simulink model "robosimulador"  (R2021b)
settings: Solver=VariableStepAuto  StartTime=0.0  StopTime=Time(length(Time))  MaxStep=1e-3  RelTol=1e-3
model workspace: external: MATLAB File /home/fabio/Desktop/Larc 2021/robosimulador_DataFile.m (data not in the file)
values from neighbouring files (symbols this model uses):
  j = length(Q)    [Cinematica_Comb.m]    (also in Cinematica_Heli_Coronal.m; Cinematica_Heli_Direta_Coronal.m; Cinematica_Heli_Sagital.m)
  Q = Qr    [Cinematica_Comb.m]
  X = zeros(1,14)    [Cinematica_Comb.m]    (also in Cinematica_Heli_Coronal.m = zeros(1,6); Cinematica_Heli_Direta_Coronal.m = zeros(1,6); Cinematica_Heli_Sagital.m = zeros(1,8))
  Y = zeros(1,14)    [Cinematica_Comb.m]    (also in Cinematica_Heli_Coronal.m = zeros(1,6); Cinematica_Heli_Direta_Coronal.m = zeros(1,6); Cinematica_Heli_Sagital.m = zeros(1,8))
  Z = zeros(1,14)    [Cinematica_Comb.m]    (also in Cinematica_Heli_Coronal.m = zeros(1,6); Cinematica_Heli_Direta_Coronal.m = zeros(1,6); Cinematica_Heli_Sagital.m = zeros(1,8))
undefined symbols (not defined in the file or in its folder): g, height_plane, plane_x, smiData, Time, Tmax, zzmp
libraries: nesl_utility x168, sm_lib x117, simulink x38, sharedutil x19, Contact_Forces_Lib x8
(part 5 of 6)

== system robosimulador/Robô/Lado Direito/Centro de Massa/Subsystem1 ==
  Mux : Mux  Inputs=3
  PS-Simulink Converter1 : nesl_utility/PS-Simulink Converter  PhysicalDomain=network_engine_domain  SubClassName=ps_output  LeftPortType=input  RightPortType=output  PseudoPeriodic=off  Frequencies=[]  Unit=m  AffineConversion=off
      settings: SourceProductBaseCode=PW,SS
  PS-Simulink Converter2 : nesl_utility/PS-Simulink Converter  PhysicalDomain=network_engine_domain  SubClassName=ps_output  LeftPortType=input  RightPortType=output  PseudoPeriodic=off  Frequencies=[]  Unit=m  AffineConversion=off
      settings: SourceProductBaseCode=PW,SS
  PS-Simulink Converter9 : nesl_utility/PS-Simulink Converter  PhysicalDomain=network_engine_domain  SubClassName=ps_output  LeftPortType=input  RightPortType=output  PseudoPeriodic=off  Frequencies=[]  Unit=m  AffineConversion=off
      settings: SourceProductBaseCode=PW,SS
  x : PMIOPort  Side=Left
  y : PMIOPort  Port=2  Side=Left
  z : PMIOPort  Port=3  Side=Left
  r : Outport  VectorParamsAs1DForOutWhenUnconnected=off
  wires:
  PS-Simulink Converter2/1 -> Mux/3
  PS-Simulink Converter1/1 -> Mux/2
  PS-Simulink Converter9/1 -> Mux/1
  Mux/1 -> r/1
  connections:
  y/RConn1 -- PS-Simulink Converter1/LConn1
  z/RConn1 -- PS-Simulink Converter2/LConn1
  x/RConn1 -- PS-Simulink Converter9/LConn1

== system robosimulador/Robô/Lado Direito/Centro de Massa/Subsystem2 ==
  Mux : Mux  Inputs=3
  PS-Simulink Converter1 : nesl_utility/PS-Simulink Converter  PhysicalDomain=network_engine_domain  SubClassName=ps_output  LeftPortType=input  RightPortType=output  PseudoPeriodic=off  Frequencies=[]  Unit=m  AffineConversion=off
      settings: SourceProductBaseCode=PW,SS
  PS-Simulink Converter2 : nesl_utility/PS-Simulink Converter  PhysicalDomain=network_engine_domain  SubClassName=ps_output  LeftPortType=input  RightPortType=output  PseudoPeriodic=off  Frequencies=[]  Unit=m  AffineConversion=off
      settings: SourceProductBaseCode=PW,SS
  PS-Simulink Converter9 : nesl_utility/PS-Simulink Converter  PhysicalDomain=network_engine_domain  SubClassName=ps_output  LeftPortType=input  RightPortType=output  PseudoPeriodic=off  Frequencies=[]  Unit=m  AffineConversion=off
      settings: SourceProductBaseCode=PW,SS
  x : PMIOPort  Side=Left
  y : PMIOPort  Port=2  Side=Left
  z : PMIOPort  Port=3  Side=Left
  r : Outport  VectorParamsAs1DForOutWhenUnconnected=off
  wires:
  Mux/1 -> r/1
  PS-Simulink Converter9/1 -> Mux/1
  PS-Simulink Converter1/1 -> Mux/2
  PS-Simulink Converter2/1 -> Mux/3
  connections:
  x/RConn1 -- PS-Simulink Converter9/LConn1
  z/RConn1 -- PS-Simulink Converter2/LConn1
  y/RConn1 -- PS-Simulink Converter1/LConn1

== system robosimulador/Robô/Lado Direito/Centro de Massa/Subsystem3 ==
  Mux : Mux  Inputs=3
  PS-Simulink Converter1 : nesl_utility/PS-Simulink Converter  PhysicalDomain=network_engine_domain  SubClassName=ps_output  LeftPortType=input  RightPortType=output  PseudoPeriodic=off  Frequencies=[]  Unit=m  AffineConversion=off
      settings: SourceProductBaseCode=PW,SS
  PS-Simulink Converter2 : nesl_utility/PS-Simulink Converter  PhysicalDomain=network_engine_domain  SubClassName=ps_output  LeftPortType=input  RightPortType=output  PseudoPeriodic=off  Frequencies=[]  Unit=m  AffineConversion=off
      settings: SourceProductBaseCode=PW,SS
  PS-Simulink Converter9 : nesl_utility/PS-Simulink Converter  PhysicalDomain=network_engine_domain  SubClassName=ps_output  LeftPortType=input  RightPortType=output  PseudoPeriodic=off  Frequencies=[]  Unit=m  AffineConversion=off
      settings: SourceProductBaseCode=PW,SS
  x : PMIOPort  Side=Left
  y : PMIOPort  Port=2  Side=Left
  z : PMIOPort  Port=3  Side=Left
  r : Outport  VectorParamsAs1DForOutWhenUnconnected=off
  wires:
  PS-Simulink Converter2/1 -> Mux/3
  PS-Simulink Converter1/1 -> Mux/2
  PS-Simulink Converter9/1 -> Mux/1
  Mux/1 -> r/1
  connections:
  y/RConn1 -- PS-Simulink Converter1/LConn1
  z/RConn1 -- PS-Simulink Converter2/LConn1
  x/RConn1 -- PS-Simulink Converter9/LConn1

== system robosimulador/Robô/Lado Direito/Centro de Massa/Subsystem4 ==
  Mux : Mux  Inputs=3
  PS-Simulink Converter1 : nesl_utility/PS-Simulink Converter  PhysicalDomain=network_engine_domain  SubClassName=ps_output  LeftPortType=input  RightPortType=output  PseudoPeriodic=off  Frequencies=[]  Unit=m  AffineConversion=off
      settings: SourceProductBaseCode=PW,SS
  PS-Simulink Converter2 : nesl_utility/PS-Simulink Converter  PhysicalDomain=network_engine_domain  SubClassName=ps_output  LeftPortType=input  RightPortType=output  PseudoPeriodic=off  Frequencies=[]  Unit=m  AffineConversion=off
      settings: SourceProductBaseCode=PW,SS
  PS-Simulink Converter9 : nesl_utility/PS-Simulink Converter  PhysicalDomain=network_engine_domain  SubClassName=ps_output  LeftPortType=input  RightPortType=output  PseudoPeriodic=off  Frequencies=[]  Unit=m  AffineConversion=off
      settings: SourceProductBaseCode=PW,SS
  x : PMIOPort  Side=Left
  y : PMIOPort  Port=2  Side=Left
  z : PMIOPort  Port=3  Side=Left
  r : Outport  VectorParamsAs1DForOutWhenUnconnected=off
  wires:
  Mux/1 -> r/1
  PS-Simulink Converter9/1 -> Mux/1
  PS-Simulink Converter1/1 -> Mux/2
  PS-Simulink Converter2/1 -> Mux/3
  connections:
  x/RConn1 -- PS-Simulink Converter9/LConn1
  z/RConn1 -- PS-Simulink Converter2/LConn1
  y/RConn1 -- PS-Simulink Converter1/LConn1

== system robosimulador/Robô/Lado Direito/Centro de Massa/Subsystem5 ==
  Mux : Mux  Inputs=3
  PS-Simulink Converter1 : nesl_utility/PS-Simulink Converter  PhysicalDomain=network_engine_domain  SubClassName=ps_output  LeftPortType=input  RightPortType=output  PseudoPeriodic=off  Frequencies=[]  Unit=m  AffineConversion=off
      settings: SourceProductBaseCode=PW,SS
  PS-Simulink Converter2 : nesl_utility/PS-Simulink Converter  PhysicalDomain=network_engine_domain  SubClassName=ps_output  LeftPortType=input  RightPortType=output  PseudoPeriodic=off  Frequencies=[]  Unit=m  AffineConversion=off
      settings: SourceProductBaseCode=PW,SS
  PS-Simulink Converter9 : nesl_utility/PS-Simulink Converter  PhysicalDomain=network_engine_domain  SubClassName=ps_output  LeftPortType=input  RightPortType=output  PseudoPeriodic=off  Frequencies=[]  Unit=m  AffineConversion=off
      settings: SourceProductBaseCode=PW,SS
  x : PMIOPort  Side=Left
  y : PMIOPort  Port=2  Side=Left
  z : PMIOPort  Port=3  Side=Left
  r : Outport  VectorParamsAs1DForOutWhenUnconnected=off
  wires:
  Mux/1 -> r/1
  PS-Simulink Converter9/1 -> Mux/1
  PS-Simulink Converter1/1 -> Mux/2
  PS-Simulink Converter2/1 -> Mux/3
  connections:
  x/RConn1 -- PS-Simulink Converter9/LConn1
  z/RConn1 -- PS-Simulink Converter2/LConn1
  y/RConn1 -- PS-Simulink Converter1/LConn1

== system robosimulador/Robô/Lado Direito/Centro de Massa/Subsystem6 ==
  Mux : Mux  Inputs=3
  PS-Simulink Converter1 : nesl_utility/PS-Simulink Converter  PhysicalDomain=network_engine_domain  SubClassName=ps_output  LeftPortType=input  RightPortType=output  PseudoPeriodic=off  Frequencies=[]  Unit=m  AffineConversion=off
      settings: SourceProductBaseCode=PW,SS
  PS-Simulink Converter2 : nesl_utility/PS-Simulink Converter  PhysicalDomain=network_engine_domain  SubClassName=ps_output  LeftPortType=input  RightPortType=output  PseudoPeriodic=off  Frequencies=[]  Unit=m  AffineConversion=off
      settings: SourceProductBaseCode=PW,SS
  PS-Simulink Converter9 : nesl_utility/PS-Simulink Converter  PhysicalDomain=network_engine_domain  SubClassName=ps_output  LeftPortType=input  RightPortType=output  PseudoPeriodic=off  Frequencies=[]  Unit=m  AffineConversion=off
      settings: SourceProductBaseCode=PW,SS
  x : PMIOPort  Side=Left
  y : PMIOPort  Port=2  Side=Left
  z : PMIOPort  Port=3  Side=Left
  r : Outport  VectorParamsAs1DForOutWhenUnconnected=off
  wires:
  PS-Simulink Converter2/1 -> Mux/3
  PS-Simulink Converter1/1 -> Mux/2
  PS-Simulink Converter9/1 -> Mux/1
  Mux/1 -> r/1
  connections:
  y/RConn1 -- PS-Simulink Converter1/LConn1
  z/RConn1 -- PS-Simulink Converter2/LConn1
  x/RConn1 -- PS-Simulink Converter9/LConn1

== system robosimulador/Robô/Lado Direito/Centro de Massa/Subsystem7 ==
  Mux : Mux  Inputs=3
  PS-Simulink Converter1 : nesl_utility/PS-Simulink Converter  PhysicalDomain=network_engine_domain  SubClassName=ps_output  LeftPortType=input  RightPortType=output  PseudoPeriodic=off  Frequencies=[]  Unit=m  AffineConversion=off
      settings: SourceProductBaseCode=PW,SS
  PS-Simulink Converter2 : nesl_utility/PS-Simulink Converter  PhysicalDomain=network_engine_domain  SubClassName=ps_output  LeftPortType=input  RightPortType=output  PseudoPeriodic=off  Frequencies=[]  Unit=m  AffineConversion=off
      settings: SourceProductBaseCode=PW,SS
  PS-Simulink Converter9 : nesl_utility/PS-Simulink Converter  PhysicalDomain=network_engine_domain  SubClassName=ps_output  LeftPortType=input  RightPortType=output  PseudoPeriodic=off  Frequencies=[]  Unit=m  AffineConversion=off
      settings: SourceProductBaseCode=PW,SS
  x : PMIOPort  Side=Left
  y : PMIOPort  Port=2  Side=Left
  z : PMIOPort  Port=3  Side=Left
  r : Outport  VectorParamsAs1DForOutWhenUnconnected=off
  wires:
  Mux/1 -> r/1
  PS-Simulink Converter9/1 -> Mux/1
  PS-Simulink Converter1/1 -> Mux/2
  PS-Simulink Converter2/1 -> Mux/3
  connections:
  x/RConn1 -- PS-Simulink Converter9/LConn1
  z/RConn1 -- PS-Simulink Converter2/LConn1
  y/RConn1 -- PS-Simulink Converter1/LConn1

== system robosimulador/Robô/Lado Direito/Centro de Massa/ZMP Ante Braco1 ==
  r : Inport
  3x3 Cross Product : sharedutil/3x3 Cross Product  aMode=aMode
      settings: SourceProductBaseCode=AE,PW,DR,MT,UV,VE
  Derivative : Derivative
  Gain1 : Gain  Gain=smiData.Solid(4).mass
  IW bat : Subsystem
  Sum : Sum
  wx : PMIOPort  Side=Left
  wy : PMIOPort  Port=2  Side=Left
  wz : PMIOPort  Port=3  Side=Left
  R : PMIOPort  Port=4  Side=Left
  Hb : Outport  VectorParamsAs1DForOutWhenUnconnected=off
  Pb : Outport  Port=2  VectorParamsAs1DForOutWhenUnconnected=off
  wires:
  IW bat/1(Iw) -> Sum/1
  r/1 -> Derivative/1, 3x3 Cross Product/1
  3x3 Cross Product/1 -> Sum/2
  Derivative/1 -> Gain1/1
  Gain1/1 -> 3x3 Cross Product/2, Pb/1
  Sum/1 -> Hb/1
  connections:
  wx/RConn1 -- IW bat/LConn1
  wy/RConn1 -- IW bat/LConn2
  IW bat/LConn3 -- wz/RConn1
  R/RConn1 -- IW bat/LConn4

== system robosimulador/Robô/Lado Direito/Centro de Massa/ZMP Braco ==
  r : Inport
  3x3 Cross Product : sharedutil/3x3 Cross Product  aMode=aMode
      settings: SourceProductBaseCode=AE,PW,DR,MT,UV,VE
  Derivative : Derivative
  Gain1 : Gain  Gain=smiData.Solid(8).mass
  IW bat : Subsystem
  Sum : Sum
  wx : PMIOPort  Side=Left
  wy : PMIOPort  Port=2  Side=Left
  wz : PMIOPort  Port=3  Side=Left
  R : PMIOPort  Port=4  Side=Left
  Hb : Outport  VectorParamsAs1DForOutWhenUnconnected=off
  Pb : Outport  Port=2  VectorParamsAs1DForOutWhenUnconnected=off
  wires:
  Sum/1 -> Hb/1
  Gain1/1 -> Pb/1, 3x3 Cross Product/2
  Derivative/1 -> Gain1/1
  3x3 Cross Product/1 -> Sum/2
  r/1 -> 3x3 Cross Product/1, Derivative/1
  IW bat/1(Iw) -> Sum/1
  connections:
  R/RConn1 -- IW bat/LConn4
  IW bat/LConn3 -- wz/RConn1
  wy/RConn1 -- IW bat/LConn2
  wx/RConn1 -- IW bat/LConn1

== system robosimulador/Robô/Lado Direito/Centro de Massa/ZMP Ombro ==
  r : Inport
  3x3 Cross Product : sharedutil/3x3 Cross Product  aMode=aMode
      settings: SourceProductBaseCode=AE,PW,DR,MT,UV,VE
  Derivative : Derivative
  Gain1 : Gain  Gain=smiData.Solid(1).mass
  IW bat : Subsystem
  Sum : Sum
  wx : PMIOPort  Side=Left
  wy : PMIOPort  Port=2  Side=Left
  wz : PMIOPort  Port=3  Side=Left
  R : PMIOPort  Port=4  Side=Left
  Hb : Outport  VectorParamsAs1DForOutWhenUnconnected=off
  Pb : Outport  Port=2  VectorParamsAs1DForOutWhenUnconnected=off
  wires:
  Sum/1 -> Hb/1
  Gain1/1 -> Pb/1, 3x3 Cross Product/2
  Derivative/1 -> Gain1/1
  3x3 Cross Product/1 -> Sum/2
  r/1 -> 3x3 Cross Product/1, Derivative/1
  IW bat/1(Iw) -> Sum/1
  connections:
  R/RConn1 -- IW bat/LConn4
  IW bat/LConn3 -- wz/RConn1
  wy/RConn1 -- IW bat/LConn2
  wx/RConn1 -- IW bat/LConn1

== system robosimulador/Robô/Lado Direito/Centro de Massa/ZMP Pe ==
  r : Inport
  3x3 Cross Product : sharedutil/3x3 Cross Product  aMode=aMode
      settings: SourceProductBaseCode=AE,PW,DR,MT,UV,VE
  Derivative : Derivative
  Gain1 : Gain  Gain=smiData.Solid(9).mass
  IW bat : Subsystem
  Sum : Sum
  wx : PMIOPort  Side=Left
  wy : PMIOPort  Port=2  Side=Left
  wz : PMIOPort  Port=3  Side=Left
  R : PMIOPort  Port=4  Side=Left
  Hb : Outport  VectorParamsAs1DForOutWhenUnconnected=off
  Pb : Outport  Port=2  VectorParamsAs1DForOutWhenUnconnected=off
  wires:
  IW bat/1(Iw) -> Sum/1
  r/1 -> Derivative/1, 3x3 Cross Product/1
  3x3 Cross Product/1 -> Sum/2
  Derivative/1 -> Gain1/1
  Gain1/1 -> Pb/1, 3x3 Cross Product/2
  Sum/1 -> Hb/1
  connections:
  wx/RConn1 -- IW bat/LConn1
  wy/RConn1 -- IW bat/LConn2
  IW bat/LConn3 -- wz/RConn1
  R/RConn1 -- IW bat/LConn4

== system robosimulador/Robô/Lado Direito/Centro de Massa/ZMP Quadril ==
  r : Inport
  3x3 Cross Product : sharedutil/3x3 Cross Product  aMode=aMode
      settings: SourceProductBaseCode=AE,PW,DR,MT,UV,VE
  Derivative : Derivative
  Gain1 : Gain  Gain=smiData.Solid(10).mass
  IW bat : Subsystem
  Sum : Sum
  wx : PMIOPort  Side=Left
  wy : PMIOPort  Port=2  Side=Left
  wz : PMIOPort  Port=3  Side=Left
  R : PMIOPort  Port=4  Side=Left
  Hb : Outport  VectorParamsAs1DForOutWhenUnconnected=off
  Pb : Outport  Port=2  VectorParamsAs1DForOutWhenUnconnected=off
  wires:
  IW bat/1(Iw) -> Sum/1
  r/1 -> Derivative/1, 3x3 Cross Product/1
  3x3 Cross Product/1 -> Sum/2
  Derivative/1 -> Gain1/1
  Gain1/1 -> Pb/1, 3x3 Cross Product/2
  Sum/1 -> Hb/1
  connections:
  wx/RConn1 -- IW bat/LConn1
  wy/RConn1 -- IW bat/LConn2
  IW bat/LConn3 -- wz/RConn1
  R/RConn1 -- IW bat/LConn4

== system robosimulador/Robô/Lado Direito/Centro de Massa/ZMP Quadril1 ==
  r : Inport
  3x3 Cross Product : sharedutil/3x3 Cross Product  aMode=aMode
      settings: SourceProductBaseCode=AE,PW,DR,MT,UV,VE
  Derivative : Derivative
  Gain1 : Gain  Gain=smiData.Solid(2).mass
  IW bat : Subsystem
  Sum : Sum
  wx : PMIOPort  Side=Left
  wy : PMIOPort  Port=2  Side=Left
  wz : PMIOPort  Port=3  Side=Left
  R : PMIOPort  Port=4  Side=Left
  Hb : Outport  VectorParamsAs1DForOutWhenUnconnected=off
  Pb : Outport  Port=2  VectorParamsAs1DForOutWhenUnconnected=off
  wires:
  Sum/1 -> Hb/1
  Gain1/1 -> 3x3 Cross Product/2, Pb/1
  Derivative/1 -> Gain1/1
  3x3 Cross Product/1 -> Sum/2
  r/1 -> 3x3 Cross Product/1, Derivative/1
  IW bat/1(Iw) -> Sum/1
  connections:
  R/RConn1 -- IW bat/LConn4
  IW bat/LConn3 -- wz/RConn1
  wy/RConn1 -- IW bat/LConn2
  wx/RConn1 -- IW bat/LConn1

== system robosimulador/Robô/Lado Direito/Centro de Massa/ZMP canela ==
  r : Inport
  3x3 Cross Product : sharedutil/3x3 Cross Product  aMode=aMode
      settings: SourceProductBaseCode=AE,PW,DR,MT,UV,VE
  Derivative : Derivative
  Gain1 : Gain  Gain=smiData.Solid(6).mass
  IW bat : Subsystem
  Sum : Sum
  wx : PMIOPort  Side=Left
  wy : PMIOPort  Port=2  Side=Left
  wz : PMIOPort  Port=3  Side=Left
  R : PMIOPort  Port=4  Side=Left
  Hb : Outport  VectorParamsAs1DForOutWhenUnconnected=off
  Pb : Outport  Port=2  VectorParamsAs1DForOutWhenUnconnected=off
  wires:
  Sum/1 -> Hb/1
  Gain1/1 -> Pb/1, 3x3 Cross Product/2
  Derivative/1 -> Gain1/1
  3x3 Cross Product/1 -> Sum/2
  r/1 -> 3x3 Cross Product/1, Derivative/1
  IW bat/1(Iw) -> Sum/1
  connections:
  R/RConn1 -- IW bat/LConn4
  IW bat/LConn3 -- wz/RConn1
  wy/RConn1 -- IW bat/LConn2
  wx/RConn1 -- IW bat/LConn1

== system robosimulador/Robô/Lado Direito/Centro de Massa/ZMP coxa ==
  r : Inport
  3x3 Cross Product : sharedutil/3x3 Cross Product  aMode=aMode
      settings: SourceProductBaseCode=AE,PW,DR,MT,UV,VE
  Derivative : Derivative
  Gain1 : Gain  Gain=smiData.Solid(5).mass
  IW bat : Subsystem
  Sum : Sum
  wx : PMIOPort  Side=Left
  wy : PMIOPort  Port=2  Side=Left
  wz : PMIOPort  Port=3  Side=Left
  R : PMIOPort  Port=4  Side=Left
  Hb : Outport  VectorParamsAs1DForOutWhenUnconnected=off
  Pb : Outport  Port=2  VectorParamsAs1DForOutWhenUnconnected=off
  wires:
  IW bat/1(Iw) -> Sum/1
  r/1 -> Derivative/1, 3x3 Cross Product/1
  3x3 Cross Product/1 -> Sum/2
  Derivative/1 -> Gain1/1
  Gain1/1 -> 3x3 Cross Product/2, Pb/1
  Sum/1 -> Hb/1
  connections:
  wx/RConn1 -- IW bat/LConn1
  wy/RConn1 -- IW bat/LConn2
  IW bat/LConn3 -- wz/RConn1
  R/RConn1 -- IW bat/LConn4

== system robosimulador/Robô/Lado Esquerdo/Centro de Massa/Subsystem ==
  Mux : Mux  Inputs=3
  PS-Simulink Converter1 : nesl_utility/PS-Simulink Converter  PhysicalDomain=network_engine_domain  SubClassName=ps_output  LeftPortType=input  RightPortType=output  PseudoPeriodic=off  Frequencies=[]  Unit=m  AffineConversion=off
      settings: SourceProductBaseCode=PW,SS
  PS-Simulink Converter2 : nesl_utility/PS-Simulink Converter  PhysicalDomain=network_engine_domain  SubClassName=ps_output  LeftPortType=input  RightPortType=output  PseudoPeriodic=off  Frequencies=[]  Unit=m  AffineConversion=off
      settings: SourceProductBaseCode=PW,SS
  PS-Simulink Converter9 : nesl_utility/PS-Simulink Converter  PhysicalDomain=network_engine_domain  SubClassName=ps_output  LeftPortType=input  RightPortType=output  PseudoPeriodic=off  Frequencies=[]  Unit=m  AffineConversion=off
      settings: SourceProductBaseCode=PW,SS
  x : PMIOPort  Side=Left
  y : PMIOPort  Port=2  Side=Left
  z : PMIOPort  Port=3  Side=Left
  r : Outport  VectorParamsAs1DForOutWhenUnconnected=off
  wires:
  Mux/1 -> r/1
  PS-Simulink Converter9/1 -> Mux/1
  PS-Simulink Converter1/1 -> Mux/2
  PS-Simulink Converter2/1 -> Mux/3
  connections:
  x/RConn1 -- PS-Simulink Converter9/LConn1
  z/RConn1 -- PS-Simulink Converter2/LConn1
  y/RConn1 -- PS-Simulink Converter1/LConn1

== system robosimulador/Robô/Lado Esquerdo/Centro de Massa/Subsystem1 ==
  Mux : Mux  Inputs=3
  PS-Simulink Converter1 : nesl_utility/PS-Simulink Converter  PhysicalDomain=network_engine_domain  SubClassName=ps_output  LeftPortType=input  RightPortType=output  PseudoPeriodic=off  Frequencies=[]  Unit=m  AffineConversion=off
      settings: SourceProductBaseCode=PW,SS
  PS-Simulink Converter2 : nesl_utility/PS-Simulink Converter  PhysicalDomain=network_engine_domain  SubClassName=ps_output  LeftPortType=input  RightPortType=output  PseudoPeriodic=off  Frequencies=[]  Unit=m  AffineConversion=off
      settings: SourceProductBaseCode=PW,SS
  PS-Simulink Converter9 : nesl_utility/PS-Simulink Converter  PhysicalDomain=network_engine_domain  SubClassName=ps_output  LeftPortType=input  RightPortType=output  PseudoPeriodic=off  Frequencies=[]  Unit=m  AffineConversion=off
      settings: SourceProductBaseCode=PW,SS
  x : PMIOPort  Side=Left
  y : PMIOPort  Port=2  Side=Left
  z : PMIOPort  Port=3  Side=Left
  r : Outport  VectorParamsAs1DForOutWhenUnconnected=off
  wires:
  PS-Simulink Converter2/1 -> Mux/3
  PS-Simulink Converter1/1 -> Mux/2
  PS-Simulink Converter9/1 -> Mux/1
  Mux/1 -> r/1
  connections:
  y/RConn1 -- PS-Simulink Converter1/LConn1
  z/RConn1 -- PS-Simulink Converter2/LConn1
  x/RConn1 -- PS-Simulink Converter9/LConn1

== system robosimulador/Robô/Lado Esquerdo/Centro de Massa/Subsystem2 ==
  Mux : Mux  Inputs=3
  PS-Simulink Converter1 : nesl_utility/PS-Simulink Converter  PhysicalDomain=network_engine_domain  SubClassName=ps_output  LeftPortType=input  RightPortType=output  PseudoPeriodic=off  Frequencies=[]  Unit=m  AffineConversion=off
      settings: SourceProductBaseCode=PW,SS
  PS-Simulink Converter2 : nesl_utility/PS-Simulink Converter  PhysicalDomain=network_engine_domain  SubClassName=ps_output  LeftPortType=input  RightPortType=output  PseudoPeriodic=off  Frequencies=[]  Unit=m  AffineConversion=off
      settings: SourceProductBaseCode=PW,SS
  PS-Simulink Converter9 : nesl_utility/PS-Simulink Converter  PhysicalDomain=network_engine_domain  SubClassName=ps_output  LeftPortType=input  RightPortType=output  PseudoPeriodic=off  Frequencies=[]  Unit=m  AffineConversion=off
      settings: SourceProductBaseCode=PW,SS
  x : PMIOPort  Side=Left
  y : PMIOPort  Port=2  Side=Left
  z : PMIOPort  Port=3  Side=Left
  r : Outport  VectorParamsAs1DForOutWhenUnconnected=off
  wires:
  Mux/1 -> r/1
  PS-Simulink Converter9/1 -> Mux/1
  PS-Simulink Converter1/1 -> Mux/2
  PS-Simulink Converter2/1 -> Mux/3
  connections:
  x/RConn1 -- PS-Simulink Converter9/LConn1
  z/RConn1 -- PS-Simulink Converter2/LConn1
  y/RConn1 -- PS-Simulink Converter1/LConn1

== system robosimulador/Robô/Lado Esquerdo/Centro de Massa/Subsystem3 ==
  Mux : Mux  Inputs=3
  PS-Simulink Converter1 : nesl_utility/PS-Simulink Converter  PhysicalDomain=network_engine_domain  SubClassName=ps_output  LeftPortType=input  RightPortType=output  PseudoPeriodic=off  Frequencies=[]  Unit=m  AffineConversion=off
      settings: SourceProductBaseCode=PW,SS
  PS-Simulink Converter2 : nesl_utility/PS-Simulink Converter  PhysicalDomain=network_engine_domain  SubClassName=ps_output  LeftPortType=input  RightPortType=output  PseudoPeriodic=off  Frequencies=[]  Unit=m  AffineConversion=off
      settings: SourceProductBaseCode=PW,SS
  PS-Simulink Converter9 : nesl_utility/PS-Simulink Converter  PhysicalDomain=network_engine_domain  SubClassName=ps_output  LeftPortType=input  RightPortType=output  PseudoPeriodic=off  Frequencies=[]  Unit=m  AffineConversion=off
      settings: SourceProductBaseCode=PW,SS
  x : PMIOPort  Side=Left
  y : PMIOPort  Port=2  Side=Left
  z : PMIOPort  Port=3  Side=Left
  r : Outport  VectorParamsAs1DForOutWhenUnconnected=off
  wires:
  PS-Simulink Converter2/1 -> Mux/3
  PS-Simulink Converter1/1 -> Mux/2
  PS-Simulink Converter9/1 -> Mux/1
  Mux/1 -> r/1
  connections:
  y/RConn1 -- PS-Simulink Converter1/LConn1
  z/RConn1 -- PS-Simulink Converter2/LConn1
  x/RConn1 -- PS-Simulink Converter9/LConn1

== system robosimulador/Robô/Lado Esquerdo/Centro de Massa/Subsystem4 ==
  Mux : Mux  Inputs=3
  PS-Simulink Converter1 : nesl_utility/PS-Simulink Converter  PhysicalDomain=network_engine_domain  SubClassName=ps_output  LeftPortType=input  RightPortType=output  PseudoPeriodic=off  Frequencies=[]  Unit=m  AffineConversion=off
      settings: SourceProductBaseCode=PW,SS
  PS-Simulink Converter2 : nesl_utility/PS-Simulink Converter  PhysicalDomain=network_engine_domain  SubClassName=ps_output  LeftPortType=input  RightPortType=output  PseudoPeriodic=off  Frequencies=[]  Unit=m  AffineConversion=off
      settings: SourceProductBaseCode=PW,SS
  PS-Simulink Converter9 : nesl_utility/PS-Simulink Converter  PhysicalDomain=network_engine_domain  SubClassName=ps_output  LeftPortType=input  RightPortType=output  PseudoPeriodic=off  Frequencies=[]  Unit=m  AffineConversion=off
      settings: SourceProductBaseCode=PW,SS
  x : PMIOPort  Side=Left
  y : PMIOPort  Port=2  Side=Left
  z : PMIOPort  Port=3  Side=Left
  r : Outport  VectorParamsAs1DForOutWhenUnconnected=off
  wires:
  Mux/1 -> r/1
  PS-Simulink Converter9/1 -> Mux/1
  PS-Simulink Converter1/1 -> Mux/2
  PS-Simulink Converter2/1 -> Mux/3
  connections:
  x/RConn1 -- PS-Simulink Converter9/LConn1
  z/RConn1 -- PS-Simulink Converter2/LConn1
  y/RConn1 -- PS-Simulink Converter1/LConn1

== system robosimulador/Robô/Lado Esquerdo/Centro de Massa/Subsystem5 ==
  Mux : Mux  Inputs=3
  PS-Simulink Converter1 : nesl_utility/PS-Simulink Converter  PhysicalDomain=network_engine_domain  SubClassName=ps_output  LeftPortType=input  RightPortType=output  PseudoPeriodic=off  Frequencies=[]  Unit=m  AffineConversion=off
      settings: SourceProductBaseCode=PW,SS
  PS-Simulink Converter2 : nesl_utility/PS-Simulink Converter  PhysicalDomain=network_engine_domain  SubClassName=ps_output  LeftPortType=input  RightPortType=output  PseudoPeriodic=off  Frequencies=[]  Unit=m  AffineConversion=off
      settings: SourceProductBaseCode=PW,SS
  PS-Simulink Converter9 : nesl_utility/PS-Simulink Converter  PhysicalDomain=network_engine_domain  SubClassName=ps_output  LeftPortType=input  RightPortType=output  PseudoPeriodic=off  Frequencies=[]  Unit=m  AffineConversion=off
      settings: SourceProductBaseCode=PW,SS
  x : PMIOPort  Side=Left
  y : PMIOPort  Port=2  Side=Left
  z : PMIOPort  Port=3  Side=Left
  r : Outport  VectorParamsAs1DForOutWhenUnconnected=off
  wires:
  Mux/1 -> r/1
  PS-Simulink Converter9/1 -> Mux/1
  PS-Simulink Converter1/1 -> Mux/2
  PS-Simulink Converter2/1 -> Mux/3
  connections:
  x/RConn1 -- PS-Simulink Converter9/LConn1
  z/RConn1 -- PS-Simulink Converter2/LConn1
  y/RConn1 -- PS-Simulink Converter1/LConn1

== system robosimulador/Robô/Lado Esquerdo/Centro de Massa/Subsystem6 ==
  Mux : Mux  Inputs=3
  PS-Simulink Converter1 : nesl_utility/PS-Simulink Converter  PhysicalDomain=network_engine_domain  SubClassName=ps_output  LeftPortType=input  RightPortType=output  PseudoPeriodic=off  Frequencies=[]  Unit=m  AffineConversion=off
      settings: SourceProductBaseCode=PW,SS
  PS-Simulink Converter2 : nesl_utility/PS-Simulink Converter  PhysicalDomain=network_engine_domain  SubClassName=ps_output  LeftPortType=input  RightPortType=output  PseudoPeriodic=off  Frequencies=[]  Unit=m  AffineConversion=off
      settings: SourceProductBaseCode=PW,SS
  PS-Simulink Converter9 : nesl_utility/PS-Simulink Converter  PhysicalDomain=network_engine_domain  SubClassName=ps_output  LeftPortType=input  RightPortType=output  PseudoPeriodic=off  Frequencies=[]  Unit=m  AffineConversion=off
      settings: SourceProductBaseCode=PW,SS
  x : PMIOPort  Side=Left
  y : PMIOPort  Port=2  Side=Left
  z : PMIOPort  Port=3  Side=Left
  r : Outport  VectorParamsAs1DForOutWhenUnconnected=off
  wires:
  PS-Simulink Converter2/1 -> Mux/3
  PS-Simulink Converter1/1 -> Mux/2
  PS-Simulink Converter9/1 -> Mux/1
  Mux/1 -> r/1
  connections:
  y/RConn1 -- PS-Simulink Converter1/LConn1
  z/RConn1 -- PS-Simulink Converter2/LConn1
  x/RConn1 -- PS-Simulink Converter9/LConn1

== system robosimulador/Robô/Lado Esquerdo/Centro de Massa/Subsystem7 ==
  Mux : Mux  Inputs=3
  PS-Simulink Converter1 : nesl_utility/PS-Simulink Converter  PhysicalDomain=network_engine_domain  SubClassName=ps_output  LeftPortType=input  RightPortType=output  PseudoPeriodic=off  Frequencies=[]  Unit=m  AffineConversion=off
      settings: SourceProductBaseCode=PW,SS
  PS-Simulink Converter2 : nesl_utility/PS-Simulink Converter  PhysicalDomain=network_engine_domain  SubClassName=ps_output  LeftPortType=input  RightPortType=output  PseudoPeriodic=off  Frequencies=[]  Unit=m  AffineConversion=off
      settings: SourceProductBaseCode=PW,SS
  PS-Simulink Converter9 : nesl_utility/PS-Simulink Converter  PhysicalDomain=network_engine_domain  SubClassName=ps_output  LeftPortType=input  RightPortType=output  PseudoPeriodic=off  Frequencies=[]  Unit=m  AffineConversion=off
      settings: SourceProductBaseCode=PW,SS
  x : PMIOPort  Side=Left
  y : PMIOPort  Port=2  Side=Left
  z : PMIOPort  Port=3  Side=Left
  r : Outport  VectorParamsAs1DForOutWhenUnconnected=off
  wires:
  Mux/1 -> r/1
  PS-Simulink Converter9/1 -> Mux/1
  PS-Simulink Converter1/1 -> Mux/2
  PS-Simulink Converter2/1 -> Mux/3
  connections:
  x/RConn1 -- PS-Simulink Converter9/LConn1
  z/RConn1 -- PS-Simulink Converter2/LConn1
  y/RConn1 -- PS-Simulink Converter1/LConn1

== system robosimulador/Robô/Lado Esquerdo/Centro de Massa/ZMP Ante Braco1 ==
  r : Inport
  3x3 Cross Product : sharedutil/3x3 Cross Product  aMode=aMode
      settings: SourceProductBaseCode=AE,PW,DR,MT,UV,VE
  Derivative : Derivative
  Gain1 : Gain  Gain=smiData.Solid(4).mass
  IW bat : Subsystem
  Sum : Sum
  wx : PMIOPort  Side=Left
  wy : PMIOPort  Port=2  Side=Left
  wz : PMIOPort  Port=3  Side=Left
  R : PMIOPort  Port=4  Side=Left
  Hb : Outport  VectorParamsAs1DForOutWhenUnconnected=off
  Pb : Outport  Port=2  VectorParamsAs1DForOutWhenUnconnected=off
  wires:
  IW bat/1(Iw) -> Sum/1
  r/1 -> Derivative/1, 3x3 Cross Product/1
  3x3 Cross Product/1 -> Sum/2
  Derivative/1 -> Gain1/1
  Gain1/1 -> 3x3 Cross Product/2, Pb/1
  Sum/1 -> Hb/1
  connections:
  wx/RConn1 -- IW bat/LConn1
  wy/RConn1 -- IW bat/LConn2
  IW bat/LConn3 -- wz/RConn1
  R/RConn1 -- IW bat/LConn4

== system robosimulador/Robô/Lado Esquerdo/Centro de Massa/ZMP Braco ==
  r : Inport
  3x3 Cross Product : sharedutil/3x3 Cross Product  aMode=aMode
      settings: SourceProductBaseCode=AE,PW,DR,MT,UV,VE
  Derivative : Derivative
  Gain1 : Gain  Gain=smiData.Solid(8).mass
  IW bat : Subsystem
  Sum : Sum
  wx : PMIOPort  Side=Left
  wy : PMIOPort  Port=2  Side=Left
  wz : PMIOPort  Port=3  Side=Left
  R : PMIOPort  Port=4  Side=Left
  Hb : Outport  VectorParamsAs1DForOutWhenUnconnected=off
  Pb : Outport  Port=2  VectorParamsAs1DForOutWhenUnconnected=off
  wires:
  Sum/1 -> Hb/1
  Gain1/1 -> Pb/1, 3x3 Cross Product/2
  Derivative/1 -> Gain1/1
  3x3 Cross Product/1 -> Sum/2
  r/1 -> 3x3 Cross Product/1, Derivative/1
  IW bat/1(Iw) -> Sum/1
  connections:
  R/RConn1 -- IW bat/LConn4
  IW bat/LConn3 -- wz/RConn1
  wy/RConn1 -- IW bat/LConn2
  wx/RConn1 -- IW bat/LConn1

== system robosimulador/Robô/Lado Esquerdo/Centro de Massa/ZMP Ombro ==
  r : Inport
  3x3 Cross Product : sharedutil/3x3 Cross Product  aMode=aMode
      settings: SourceProductBaseCode=AE,PW,DR,MT,UV,VE
  Derivative : Derivative
  Gain1 : Gain  Gain=smiData.Solid(1).mass
  IW bat : Subsystem
  Sum : Sum
  wx : PMIOPort  Side=Left
  wy : PMIOPort  Port=2  Side=Left
  wz : PMIOPort  Port=3  Side=Left
  R : PMIOPort  Port=4  Side=Left
  Hb : Outport  VectorParamsAs1DForOutWhenUnconnected=off
  Pb : Outport  Port=2  VectorParamsAs1DForOutWhenUnconnected=off
  wires:
  Sum/1 -> Hb/1
  Gain1/1 -> Pb/1, 3x3 Cross Product/2
  Derivative/1 -> Gain1/1
  3x3 Cross Product/1 -> Sum/2
  r/1 -> 3x3 Cross Product/1, Derivative/1
  IW bat/1(Iw) -> Sum/1
  connections:
  R/RConn1 -- IW bat/LConn4
  IW bat/LConn3 -- wz/RConn1
  wy/RConn1 -- IW bat/LConn2
  wx/RConn1 -- IW bat/LConn1

== system robosimulador/Robô/Lado Esquerdo/Centro de Massa/ZMP Pe ==
  r : Inport
  3x3 Cross Product : sharedutil/3x3 Cross Product  aMode=aMode
      settings: SourceProductBaseCode=AE,PW,DR,MT,UV,VE
  Derivative : Derivative
  Gain1 : Gain  Gain=smiData.Solid(9).mass
  IW bat : Subsystem
  Sum : Sum
  wx : PMIOPort  Side=Left
  wy : PMIOPort  Port=2  Side=Left
  wz : PMIOPort  Port=3  Side=Left
  R : PMIOPort  Port=4  Side=Left
  Hb : Outport  VectorParamsAs1DForOutWhenUnconnected=off
  Pb : Outport  Port=2  VectorParamsAs1DForOutWhenUnconnected=off
  wires:
  IW bat/1(Iw) -> Sum/1
  r/1 -> Derivative/1, 3x3 Cross Product/1
  3x3 Cross Product/1 -> Sum/2
  Derivative/1 -> Gain1/1
  Gain1/1 -> Pb/1, 3x3 Cross Product/2
  Sum/1 -> Hb/1
  connections:
  wx/RConn1 -- IW bat/LConn1
  wy/RConn1 -- IW bat/LConn2
  IW bat/LConn3 -- wz/RConn1
  R/RConn1 -- IW bat/LConn4

== system robosimulador/Robô/Lado Esquerdo/Centro de Massa/ZMP Quadril ==
  r : Inport
  3x3 Cross Product : sharedutil/3x3 Cross Product  aMode=aMode
      settings: SourceProductBaseCode=AE,PW,DR,MT,UV,VE
  Derivative : Derivative
  Gain1 : Gain  Gain=smiData.Solid(10).mass
  IW bat : Subsystem
  Sum : Sum
  wx : PMIOPort  Side=Left
  wy : PMIOPort  Port=2  Side=Left
  wz : PMIOPort  Port=3  Side=Left
  R : PMIOPort  Port=4  Side=Left
  Hb : Outport  VectorParamsAs1DForOutWhenUnconnected=off
  Pb : Outport  Port=2  VectorParamsAs1DForOutWhenUnconnected=off
  wires:
  IW bat/1(Iw) -> Sum/1
  r/1 -> Derivative/1, 3x3 Cross Product/1
  3x3 Cross Product/1 -> Sum/2
  Derivative/1 -> Gain1/1
  Gain1/1 -> Pb/1, 3x3 Cross Product/2
  Sum/1 -> Hb/1
  connections:
  wx/RConn1 -- IW bat/LConn1
  wy/RConn1 -- IW bat/LConn2
  IW bat/LConn3 -- wz/RConn1
  R/RConn1 -- IW bat/LConn4

== system robosimulador/Robô/Lado Esquerdo/Centro de Massa/ZMP Quadril1 ==
  r : Inport
  3x3 Cross Product : sharedutil/3x3 Cross Product  aMode=aMode
      settings: SourceProductBaseCode=AE,PW,DR,MT,UV,VE
  Derivative : Derivative
  Gain1 : Gain  Gain=smiData.Solid(2).mass
  IW bat : Subsystem
  Sum : Sum
  wx : PMIOPort  Side=Left
  wy : PMIOPort  Port=2  Side=Left
  wz : PMIOPort  Port=3  Side=Left
  R : PMIOPort  Port=4  Side=Left
  Hb : Outport  VectorParamsAs1DForOutWhenUnconnected=off
  Pb : Outport  Port=2  VectorParamsAs1DForOutWhenUnconnected=off
  wires:
  Sum/1 -> Hb/1
  Gain1/1 -> 3x3 Cross Product/2, Pb/1
  Derivative/1 -> Gain1/1
  3x3 Cross Product/1 -> Sum/2
  r/1 -> 3x3 Cross Product/1, Derivative/1
  IW bat/1(Iw) -> Sum/1
  connections:
  R/RConn1 -- IW bat/LConn4
  IW bat/LConn3 -- wz/RConn1
  wy/RConn1 -- IW bat/LConn2
  wx/RConn1 -- IW bat/LConn1

== system robosimulador/Robô/Lado Esquerdo/Centro de Massa/ZMP canela ==
  r : Inport
  3x3 Cross Product : sharedutil/3x3 Cross Product  aMode=aMode
      settings: SourceProductBaseCode=AE,PW,DR,MT,UV,VE
  Derivative : Derivative
  Gain1 : Gain  Gain=smiData.Solid(6).mass
  IW bat : Subsystem
  Sum : Sum
  wx : PMIOPort  Side=Left
  wy : PMIOPort  Port=2  Side=Left
  wz : PMIOPort  Port=3  Side=Left
  R : PMIOPort  Port=4  Side=Left
  Hb : Outport  VectorParamsAs1DForOutWhenUnconnected=off
  Pb : Outport  Port=2  VectorParamsAs1DForOutWhenUnconnected=off
  wires:
  Sum/1 -> Hb/1
  Gain1/1 -> Pb/1, 3x3 Cross Product/2
  Derivative/1 -> Gain1/1
  3x3 Cross Product/1 -> Sum/2
  r/1 -> 3x3 Cross Product/1, Derivative/1
  IW bat/1(Iw) -> Sum/1
  connections:
  R/RConn1 -- IW bat/LConn4
  IW bat/LConn3 -- wz/RConn1
  wy/RConn1 -- IW bat/LConn2
  wx/RConn1 -- IW bat/LConn1

== system robosimulador/Robô/Lado Esquerdo/Centro de Massa/ZMP coxa ==
  r : Inport
  3x3 Cross Product : sharedutil/3x3 Cross Product  aMode=aMode
      settings: SourceProductBaseCode=AE,PW,DR,MT,UV,VE
  Derivative : Derivative
  Gain1 : Gain  Gain=smiData.Solid(5).mass
  IW bat : Subsystem
  Sum : Sum
  wx : PMIOPort  Side=Left
  wy : PMIOPort  Port=2  Side=Left
  wz : PMIOPort  Port=3  Side=Left
  R : PMIOPort  Port=4  Side=Left
  Hb : Outport  VectorParamsAs1DForOutWhenUnconnected=off
  Pb : Outport  Port=2  VectorParamsAs1DForOutWhenUnconnected=off
  wires:
  IW bat/1(Iw) -> Sum/1
  r/1 -> Derivative/1, 3x3 Cross Product/1
  3x3 Cross Product/1 -> Sum/2
  Derivative/1 -> Gain1/1
  Gain1/1 -> 3x3 Cross Product/2, Pb/1
  Sum/1 -> Hb/1
  connections:
  wx/RConn1 -- IW bat/LConn1
  wy/RConn1 -- IW bat/LConn2
  IW bat/LConn3 -- wz/RConn1
  R/RConn1 -- IW bat/LConn4

== system robosimulador/Robô/Torso/CoM e ZMP Superior/ZMP Torso ==
  r : Inport
  3x3 Cross Product : sharedutil/3x3 Cross Product  aMode=aMode
      settings: SourceProductBaseCode=AE,PW,DR,MT,UV,VE
  Derivative : Derivative
  Gain1 : Gain  Gain=smiData.Solid(7).mass
  IW bat : Subsystem
  Sum : Sum
  wx : PMIOPort  Side=Left
  wy : PMIOPort  Port=2  Side=Left
  wz : PMIOPort  Port=3  Side=Left
  R : PMIOPort  Port=4  Side=Left
  Hb : Outport  VectorParamsAs1DForOutWhenUnconnected=off
  Pb : Outport  Port=2  VectorParamsAs1DForOutWhenUnconnected=off
  wires:
  Sum/1 -> Hb/1
  Gain1/1 -> Pb/1, 3x3 Cross Product/2
  Derivative/1 -> Gain1/1
  3x3 Cross Product/1 -> Sum/2
  r/1 -> 3x3 Cross Product/1, Derivative/1
  IW bat/1(Iw) -> Sum/1
  connections:
  R/RConn1 -- IW bat/LConn4
  IW bat/LConn3 -- wz/RConn1
  wy/RConn1 -- IW bat/LConn2
  wx/RConn1 -- IW bat/LConn1

== system robosimulador/Robô/Torso/CoM e ZMP Superior/ZMP cabeça  ==
  r : Inport
  3x3 Cross Product : sharedutil/3x3 Cross Product  aMode=aMode
      settings: SourceProductBaseCode=AE,PW,DR,MT,UV,VE
  Derivative : Derivative
  Gain1 : Gain  Gain=smiData.Solid(3).mass
  IW cab : Subsystem
  Sum : Sum
  wx : PMIOPort  Side=Left
  wy : PMIOPort  Port=2  Side=Left
  wz : PMIOPort  Port=3  Side=Left
  R : PMIOPort  Port=4  Side=Left
  Hb : Outport  VectorParamsAs1DForOutWhenUnconnected=off
  Pb : Outport  Port=2  VectorParamsAs1DForOutWhenUnconnected=off
  wires:
  IW cab/1(Iw) -> Sum/1
  r/1 -> Derivative/1, 3x3 Cross Product/1
  3x3 Cross Product/1 -> Sum/2
  Derivative/1 -> Gain1/1
  Gain1/1 -> 3x3 Cross Product/2, Pb/1
  Sum/1 -> Hb/1
  connections:
  wx/RConn1 -- IW cab/LConn1
  wy/RConn1 -- IW cab/LConn2
  IW cab/LConn3 -- wz/RConn1
  R/RConn1 -- IW cab/LConn4

== system robosimulador/Robô/Torso/CoM e ZMP Superior/ZMP cabeça 1 ==
  r : Inport
  3x3 Cross Product : sharedutil/3x3 Cross Product  aMode=aMode
      settings: SourceProductBaseCode=AE,PW,DR,MT,UV,VE
  Derivative : Derivative
  Gain1 : Gain  Gain=smiData.Solid(11).mass
  IW cab : Subsystem
  Sum : Sum
  wx : PMIOPort  Side=Left
  wy : PMIOPort  Port=2  Side=Left
  wz : PMIOPort  Port=3  Side=Left
  R : PMIOPort  Port=4  Side=Left
  Hb : Outport  VectorParamsAs1DForOutWhenUnconnected=off
  Pb : Outport  Port=2  VectorParamsAs1DForOutWhenUnconnected=off
  wires:
  Sum/1 -> Hb/1
  Gain1/1 -> Pb/1, 3x3 Cross Product/2
  Derivative/1 -> Gain1/1
  3x3 Cross Product/1 -> Sum/2
  r/1 -> 3x3 Cross Product/1, Derivative/1
  IW cab/1(Iw) -> Sum/1
  connections:
  R/RConn1 -- IW cab/LConn4
  IW cab/LConn3 -- wz/RConn1
  wy/RConn1 -- IW cab/LConn2
  wx/RConn1 -- IW cab/LConn1

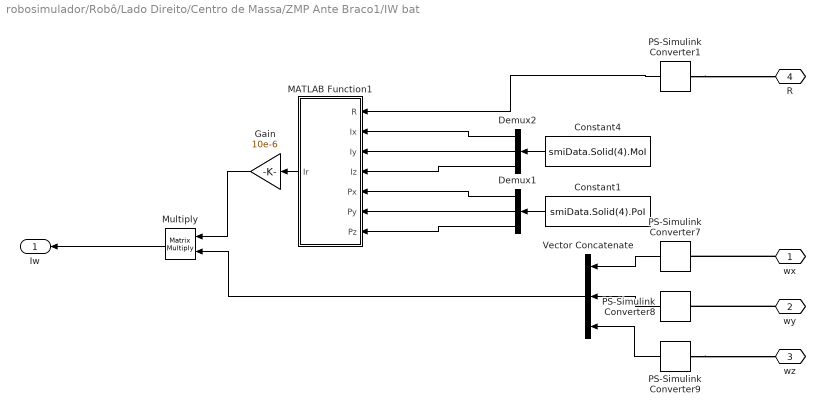
== system robosimulador/Robô/Lado Direito/Centro de Massa/ZMP Ante Braco1/IW bat ==
  Constant1 : Constant  Value=smiData.Solid(4).PoI
  Constant4 : Constant  Value=smiData.Solid(4).MoI
  Demux1 : Demux  Outputs=3
  Demux2 : Demux  Outputs=3
  Gain : Gain  Gain=10e-6
  MATLAB Function1 : MATLAB Function  TreatAsAtomicUnit=on
  Multiply : Product  Multiplication=Matrix(*)
  PS-Simulink Converter1 : nesl_utility/PS-Simulink Converter  PhysicalDomain=network_engine_domain  SubClassName=ps_output  LeftPortType=input  RightPortType=output  PseudoPeriodic=off  Frequencies=[]  Unit=rad  AffineConversion=off
      settings: SourceProductBaseCode=PW,SS
  PS-Simulink Converter7 : nesl_utility/PS-Simulink Converter  PhysicalDomain=network_engine_domain  SubClassName=ps_output  LeftPortType=input  RightPortType=output  PseudoPeriodic=off  Frequencies=[]  Unit=rad/s  AffineConversion=off
      settings: SourceProductBaseCode=PW,SS
  PS-Simulink Converter8 : nesl_utility/PS-Simulink Converter  PhysicalDomain=network_engine_domain  SubClassName=ps_output  LeftPortType=input  RightPortType=output  PseudoPeriodic=off  Frequencies=[]  Unit=rad/s  AffineConversion=off
      settings: SourceProductBaseCode=PW,SS
  PS-Simulink Converter9 : nesl_utility/PS-Simulink Converter  PhysicalDomain=network_engine_domain  SubClassName=ps_output  LeftPortType=input  RightPortType=output  PseudoPeriodic=off  Frequencies=[]  Unit=rad/s  AffineConversion=off
      settings: SourceProductBaseCode=PW,SS
  Vector Concatenate : Concatenate  NumInputs=3
  wx : PMIOPort  Side=Left
  wy : PMIOPort  Port=2  Side=Left
  wz : PMIOPort  Port=3  Side=Left
  R : PMIOPort  Port=4  Side=Left
  Iw : Outport  VectorParamsAs1DForOutWhenUnconnected=off
  wires:
  Demux2/1 -> MATLAB Function1/2(Ix)
  Demux2/3 -> MATLAB Function1/4(Iz)
  PS-Simulink Converter7/1 -> Vector Concatenate/1
  Demux1/1 -> MATLAB Function1/5(Px)
  Demux1/2 -> MATLAB Function1/6(Py)
  Constant1/1 -> Demux1/1
  PS-Simulink Converter8/1 -> Vector Concatenate/2
  Vector Concatenate/1 -> Multiply/2
  PS-Simulink Converter9/1 -> Vector Concatenate/3
  MATLAB Function1/1(Ir) -> Gain/1
  Multiply/1 -> Iw/1
  Demux2/2 -> MATLAB Function1/3(Iy)
  Demux1/3 -> MATLAB Function1/7(Pz)
  Gain/1 -> Multiply/1
  Constant4/1 -> Demux2/1
  PS-Simulink Converter1/1 -> MATLAB Function1/1(R)
  connections:
  PS-Simulink Converter9/LConn1 -- wz/RConn1
  wx/RConn1 -- PS-Simulink Converter7/LConn1
  wy/RConn1 -- PS-Simulink Converter8/LConn1
  PS-Simulink Converter1/LConn1 -- R/RConn1

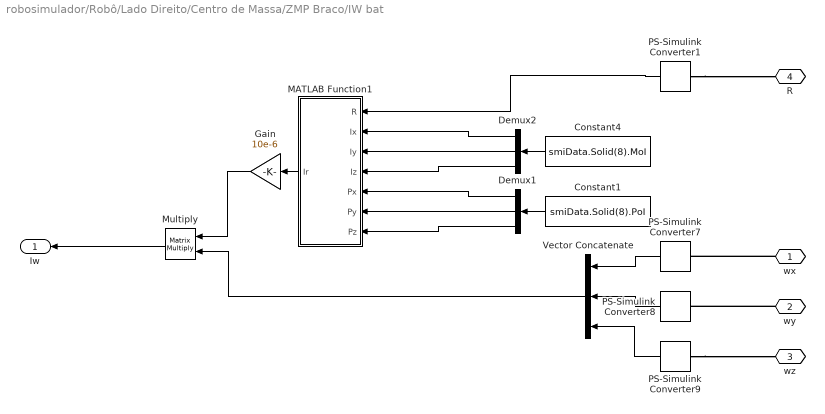
== system robosimulador/Robô/Lado Direito/Centro de Massa/ZMP Braco/IW bat ==
  Constant1 : Constant  Value=smiData.Solid(8).PoI
  Constant4 : Constant  Value=smiData.Solid(8).MoI
  Demux1 : Demux  Outputs=3
  Demux2 : Demux  Outputs=3
  Gain : Gain  Gain=10e-6
  MATLAB Function1 : MATLAB Function  TreatAsAtomicUnit=on
  Multiply : Product  Multiplication=Matrix(*)
  PS-Simulink Converter1 : nesl_utility/PS-Simulink Converter  PhysicalDomain=network_engine_domain  SubClassName=ps_output  LeftPortType=input  RightPortType=output  PseudoPeriodic=off  Frequencies=[]  Unit=rad  AffineConversion=off
      settings: SourceProductBaseCode=PW,SS
  PS-Simulink Converter7 : nesl_utility/PS-Simulink Converter  PhysicalDomain=network_engine_domain  SubClassName=ps_output  LeftPortType=input  RightPortType=output  PseudoPeriodic=off  Frequencies=[]  Unit=rad/s  AffineConversion=off
      settings: SourceProductBaseCode=PW,SS
  PS-Simulink Converter8 : nesl_utility/PS-Simulink Converter  PhysicalDomain=network_engine_domain  SubClassName=ps_output  LeftPortType=input  RightPortType=output  PseudoPeriodic=off  Frequencies=[]  Unit=rad/s  AffineConversion=off
      settings: SourceProductBaseCode=PW,SS
  PS-Simulink Converter9 : nesl_utility/PS-Simulink Converter  PhysicalDomain=network_engine_domain  SubClassName=ps_output  LeftPortType=input  RightPortType=output  PseudoPeriodic=off  Frequencies=[]  Unit=rad/s  AffineConversion=off
      settings: SourceProductBaseCode=PW,SS
  Vector Concatenate : Concatenate  NumInputs=3
  wx : PMIOPort  Side=Left
  wy : PMIOPort  Port=2  Side=Left
  wz : PMIOPort  Port=3  Side=Left
  R : PMIOPort  Port=4  Side=Left
  Iw : Outport  VectorParamsAs1DForOutWhenUnconnected=off
  wires:
  PS-Simulink Converter1/1 -> MATLAB Function1/1(R)
  Constant4/1 -> Demux2/1
  Gain/1 -> Multiply/1
  Demux1/3 -> MATLAB Function1/7(Pz)
  Demux2/2 -> MATLAB Function1/3(Iy)
  Multiply/1 -> Iw/1
  MATLAB Function1/1(Ir) -> Gain/1
  PS-Simulink Converter9/1 -> Vector Concatenate/3
  Vector Concatenate/1 -> Multiply/2
  PS-Simulink Converter8/1 -> Vector Concatenate/2
  Constant1/1 -> Demux1/1
  Demux1/2 -> MATLAB Function1/6(Py)
  Demux1/1 -> MATLAB Function1/5(Px)
  PS-Simulink Converter7/1 -> Vector Concatenate/1
  Demux2/3 -> MATLAB Function1/4(Iz)
  Demux2/1 -> MATLAB Function1/2(Ix)
  connections:
  PS-Simulink Converter1/LConn1 -- R/RConn1
  wy/RConn1 -- PS-Simulink Converter8/LConn1
  wx/RConn1 -- PS-Simulink Converter7/LConn1
  PS-Simulink Converter9/LConn1 -- wz/RConn1

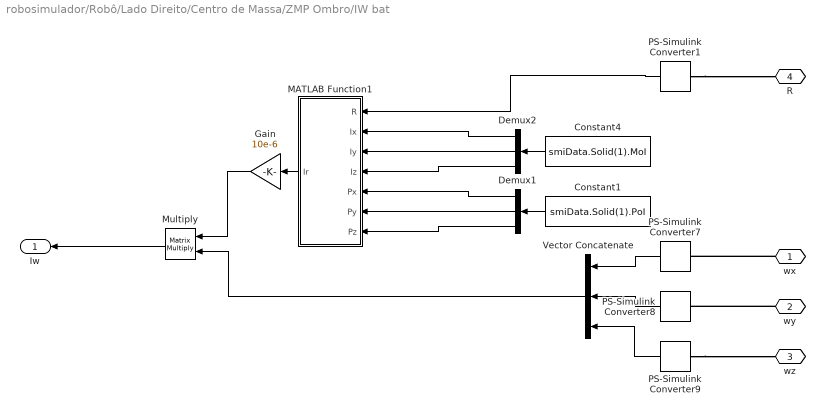
== system robosimulador/Robô/Lado Direito/Centro de Massa/ZMP Ombro/IW bat ==
  Constant1 : Constant  Value=smiData.Solid(1).PoI
  Constant4 : Constant  Value=smiData.Solid(1).MoI
  Demux1 : Demux  Outputs=3
  Demux2 : Demux  Outputs=3
  Gain : Gain  Gain=10e-6
  MATLAB Function1 : MATLAB Function  TreatAsAtomicUnit=on
  Multiply : Product  Multiplication=Matrix(*)
  PS-Simulink Converter1 : nesl_utility/PS-Simulink Converter  PhysicalDomain=network_engine_domain  SubClassName=ps_output  LeftPortType=input  RightPortType=output  PseudoPeriodic=off  Frequencies=[]  Unit=rad  AffineConversion=off
      settings: SourceProductBaseCode=PW,SS
  PS-Simulink Converter7 : nesl_utility/PS-Simulink Converter  PhysicalDomain=network_engine_domain  SubClassName=ps_output  LeftPortType=input  RightPortType=output  PseudoPeriodic=off  Frequencies=[]  Unit=rad/s  AffineConversion=off
      settings: SourceProductBaseCode=PW,SS
  PS-Simulink Converter8 : nesl_utility/PS-Simulink Converter  PhysicalDomain=network_engine_domain  SubClassName=ps_output  LeftPortType=input  RightPortType=output  PseudoPeriodic=off  Frequencies=[]  Unit=rad/s  AffineConversion=off
      settings: SourceProductBaseCode=PW,SS
  PS-Simulink Converter9 : nesl_utility/PS-Simulink Converter  PhysicalDomain=network_engine_domain  SubClassName=ps_output  LeftPortType=input  RightPortType=output  PseudoPeriodic=off  Frequencies=[]  Unit=rad/s  AffineConversion=off
      settings: SourceProductBaseCode=PW,SS
  Vector Concatenate : Concatenate  NumInputs=3
  wx : PMIOPort  Side=Left
  wy : PMIOPort  Port=2  Side=Left
  wz : PMIOPort  Port=3  Side=Left
  R : PMIOPort  Port=4  Side=Left
  Iw : Outport  VectorParamsAs1DForOutWhenUnconnected=off
  wires:
  PS-Simulink Converter1/1 -> MATLAB Function1/1(R)
  Constant4/1 -> Demux2/1
  Gain/1 -> Multiply/1
  Demux1/3 -> MATLAB Function1/7(Pz)
  Demux2/2 -> MATLAB Function1/3(Iy)
  Multiply/1 -> Iw/1
  MATLAB Function1/1(Ir) -> Gain/1
  PS-Simulink Converter9/1 -> Vector Concatenate/3
  Vector Concatenate/1 -> Multiply/2
  PS-Simulink Converter8/1 -> Vector Concatenate/2
  Constant1/1 -> Demux1/1
  Demux1/2 -> MATLAB Function1/6(Py)
  Demux1/1 -> MATLAB Function1/5(Px)
  PS-Simulink Converter7/1 -> Vector Concatenate/1
  Demux2/3 -> MATLAB Function1/4(Iz)
  Demux2/1 -> MATLAB Function1/2(Ix)
  connections:
  PS-Simulink Converter1/LConn1 -- R/RConn1
  wy/RConn1 -- PS-Simulink Converter8/LConn1
  wx/RConn1 -- PS-Simulink Converter7/LConn1
  PS-Simulink Converter9/LConn1 -- wz/RConn1

== system robosimulador/Robô/Lado Direito/Centro de Massa/ZMP Pe/IW bat ==
  Constant1 : Constant  Value=smiData.Solid(9).PoI
  Constant4 : Constant  Value=smiData.Solid(9).MoI
  Demux1 : Demux  Outputs=3
  Demux2 : Demux  Outputs=3
  Gain : Gain  Gain=10e-6
  MATLAB Function1 : MATLAB Function  TreatAsAtomicUnit=on
  Multiply : Product  Multiplication=Matrix(*)
  PS-Simulink Converter1 : nesl_utility/PS-Simulink Converter  PhysicalDomain=network_engine_domain  SubClassName=ps_output  LeftPortType=input  RightPortType=output  PseudoPeriodic=off  Frequencies=[]  Unit=rad  AffineConversion=off
      settings: SourceProductBaseCode=PW,SS
  PS-Simulink Converter7 : nesl_utility/PS-Simulink Converter  PhysicalDomain=network_engine_domain  SubClassName=ps_output  LeftPortType=input  RightPortType=output  PseudoPeriodic=off  Frequencies=[]  Unit=rad/s  AffineConversion=off
      settings: SourceProductBaseCode=PW,SS
  PS-Simulink Converter8 : nesl_utility/PS-Simulink Converter  PhysicalDomain=network_engine_domain  SubClassName=ps_output  LeftPortType=input  RightPortType=output  PseudoPeriodic=off  Frequencies=[]  Unit=rad/s  AffineConversion=off
      settings: SourceProductBaseCode=PW,SS
  PS-Simulink Converter9 : nesl_utility/PS-Simulink Converter  PhysicalDomain=network_engine_domain  SubClassName=ps_output  LeftPortType=input  RightPortType=output  PseudoPeriodic=off  Frequencies=[]  Unit=rad/s  AffineConversion=off
      settings: SourceProductBaseCode=PW,SS
  Vector Concatenate : Concatenate  NumInputs=3
  wx : PMIOPort  Side=Left
  wy : PMIOPort  Port=2  Side=Left
  wz : PMIOPort  Port=3  Side=Left
  R : PMIOPort  Port=4  Side=Left
  Iw : Outport  VectorParamsAs1DForOutWhenUnconnected=off
  wires:
  Demux2/1 -> MATLAB Function1/2(Ix)
  Demux2/3 -> MATLAB Function1/4(Iz)
  PS-Simulink Converter7/1 -> Vector Concatenate/1
  Demux1/1 -> MATLAB Function1/5(Px)
  Demux1/2 -> MATLAB Function1/6(Py)
  Constant1/1 -> Demux1/1
  PS-Simulink Converter8/1 -> Vector Concatenate/2
  Vector Concatenate/1 -> Multiply/2
  PS-Simulink Converter9/1 -> Vector Concatenate/3
  MATLAB Function1/1(Ir) -> Gain/1
  Multiply/1 -> Iw/1
  Demux2/2 -> MATLAB Function1/3(Iy)
  Demux1/3 -> MATLAB Function1/7(Pz)
  Gain/1 -> Multiply/1
  Constant4/1 -> Demux2/1
  PS-Simulink Converter1/1 -> MATLAB Function1/1(R)
  connections:
  PS-Simulink Converter9/LConn1 -- wz/RConn1
  wx/RConn1 -- PS-Simulink Converter7/LConn1
  wy/RConn1 -- PS-Simulink Converter8/LConn1
  PS-Simulink Converter1/LConn1 -- R/RConn1
